simulink model "untitled"  (R2020a)
settings: Solver=VariableStepAuto  StartTime=0.0  StopTime=10.0  RelTol=1e-3
InitFcn:
  | r = 5;
  | c = 0.3;
  | u = 5;
settings Model: Creator=muham  LastModifiedBy=muham

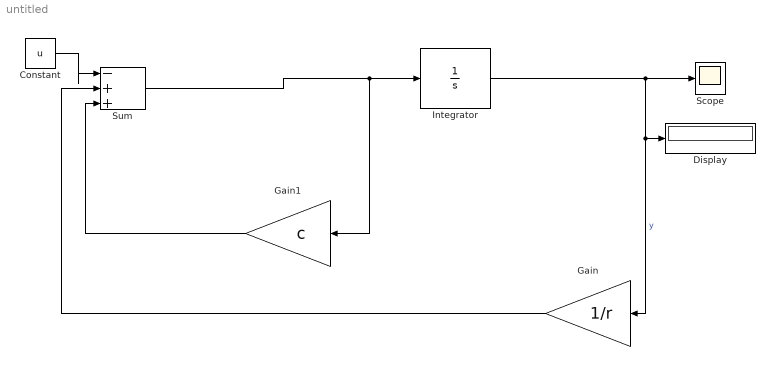
== system untitled ==
  Constant : Constant  Value=u
  Display : Display
  Gain : Gain  Gain=1/r
  Gain1 : Gain  Gain=c
  Integrator : Integrator
  Scope : Scope
  Sum : Sum  Inputs=|-++
  wires:
  Sum/1 -> Gain1/1, Integrator/1
  Integrator/1 -> Display/1, Gain/1, Scope/1  "y"
  Gain1/1 -> Sum/3
  Gain/1 -> Sum/2
  Constant/1 -> Sum/1
